simulink model "ThdRwLtStRclCmdSrvCal"  (R2024b)
settings: Solver=FixedStepDiscrete  StartTime=0.0  StopTime=10.0  FixedStep=0.01  RelTol=1e-3
undefined symbols (not defined in the file or in its folder): KeSMSwPosInvalidVal_Val, PowerMode1
settings Model: Creator=sn2xws  LastModifiedBy=sn55gm
settings SolverCC: AlgebraicLoopSolver=TrustRegion
settings DataIOCC: SaveFormat=StructureWithTime  ReturnWorkspaceOutputs=off
settings OptimizationCC: DefaultParameterBehavior=Inlined  EnhancedBackFolding=on  PassReuseOutputArgsAs=Individual arguments  ZeroExternalMemoryAtStartup=off  ZeroInternalMemoryAtStartup=off  OptimizeBlockOrder=speed  DifferentSizesBufferReuse=on  OptimizationCustomize=off  EfficientTunableParamExpr=on
settings DebuggingCC: ParameterTunabilityLossMsg=error  UnconnectedInputMsg=warning  UnconnectedOutputMsg=warning  UnconnectedLineMsg=warning  ArithmeticOperatorsInVariantConditions=warning
settings ModelReferenceCC: EnableRefExpFcnMdlSchedulingChecks=on  ModelReferenceNumInstancesAllowed=Single
settings SFSimCC: MATLABDynamicMemAlloc=off  CustomCodeUndefinedFunction=UseInterfaceOnly
settings RTWCC: Description=AUTOSAR  SystemTargetFile=autosar.tlc  GenCodeOnly=on  TemplateMakefile=ert_default_tmf  GenerateReport=on  IncludeHyperlinkInReport=on  LaunchReport=on  DataTypeReplacement=CDataTypesFixedWidth  GenerateTraceInfo=on  GenerateTraceReport=on  GenerateTraceReportSl=on  GenerateTraceReportSf=on  GenerateTraceReportEml=on  GenerateCodeMetricsReport=on  GPUComputeCapability=3.5
settings CodeAppCC: ForceParamTrailComments=on  IgnoreCustomStorageClasses=off  OperatorAnnotations=on  SimulinkDataObjDesc=on  SFDataObjDesc=on  InsertBlockDesc=on
settings STFCustomTargetCC: TargetLangStandard=C99 (ISO)  MultiwordLength=256  ParMdlRefBuildCompliant=on  CompOptLevelCompliant=on  IncludeMdlTerminateFcn=off  CombineOutputUpdateFcns=on  SuppressErrorStatus=on  ERTCustomFileBanners=on  SupportNonFinite=off  SupportComplex=off  SupportContinuousTime=off  SupportNonInlinedSFcns=off  RemoveResetFunc=on  MATLABClassNameForMDSCustomization=Simulink.SoftwareTarget.ERTCustomization  AutosarCompliant=on  UseToolchainInfoCompliant=on  LookupTableObjectStructAxisOrder=2,1,3,4,...  LUTObjectStructOrderEvenSpacing=Size,Table,Breakpoints  SystemTargetFile=autosar.tlc
settings ERTTargetCC: TargetLangStandard=C99 (ISO)  ConcurrentExecutionCompliant=off  IncludeMdlTerminateFcn=off  SuppressErrorStatus=on  SupportNonFinite=off  SupportComplex=off  ModelStepFunctionPrototypeControlCompliant=off  CPPClassGenCompliant=off  AutosarCompliant=on  LookupTableObjectStructAxisOrder=2,1,3,4,...  LUTObjectStructOrderEvenSpacing=Size,Table,Breakpoints  ERTCustomFileTemplate=example_file_process.tlc  ERTFilePackagingFormat=Compact  BooleanTrueId=TRUE  BooleanFalseId=FALSE  DynamicArrayContainerType=coder::array

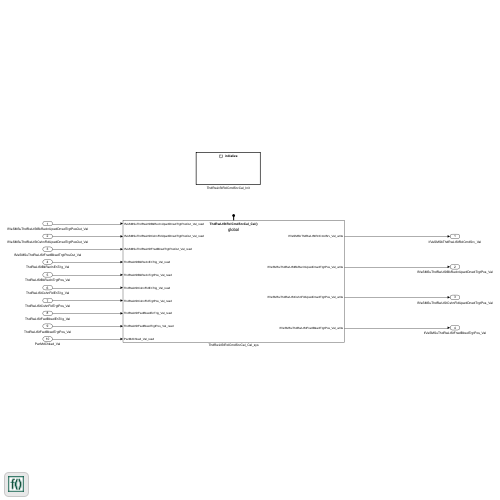
[thumbnail: Simulink's stored preview of the top-level diagram]
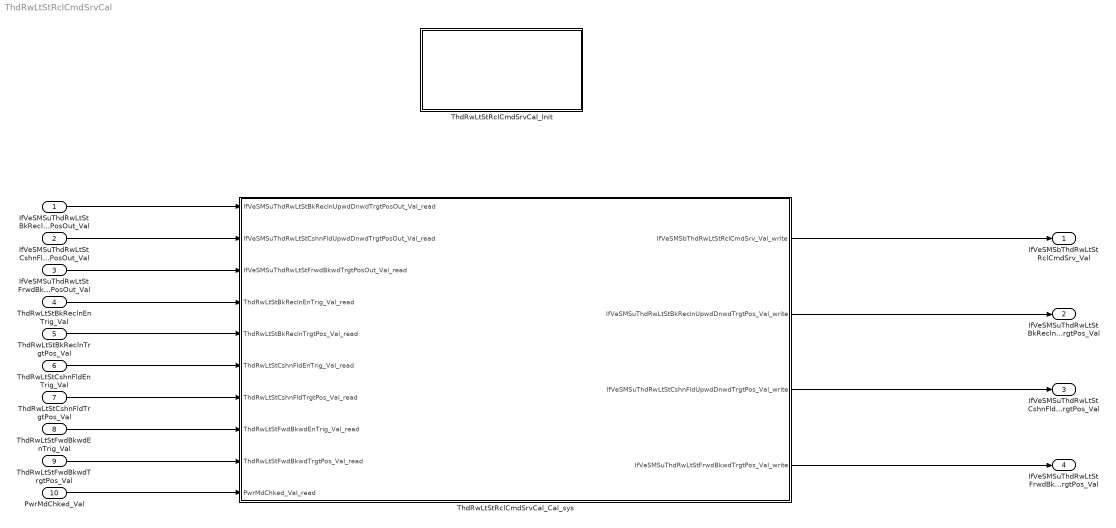
== system ThdRwLtStRclCmdSrvCal ==
  IfVeSMSuThdRwLtStBkReclnUpwdDnwdTrgtPosOut_Val : Inport  OutDataTypeStr=boolean  PortDimensions=1
  IfVeSMSuThdRwLtStCshnFldUpwdDnwdTrgtPosOut_Val : Inport  Port=2  OutDataTypeStr=boolean  PortDimensions=1
  IfVeSMSuThdRwLtStFrwdBkwdTrgtPosOut_Val : Inport  Port=3  OutDataTypeStr=boolean  PortDimensions=1
  ThdRwLtStBkReclnEnTrig_Val : Inport  Port=4  OutDataTypeStr=boolean  PortDimensions=1
  ThdRwLtStBkReclnTrgtPos_Val : Inport  Port=5  OutDataTypeStr=uint16  PortDimensions=1
  ThdRwLtStCshnFldEnTrig_Val : Inport  Port=6  OutDataTypeStr=boolean  PortDimensions=1
  ThdRwLtStCshnFldTrgtPos_Val : Inport  Port=7  OutDataTypeStr=uint16  PortDimensions=1
  ThdRwLtStFwdBkwdEnTrig_Val : Inport  Port=8  OutDataTypeStr=boolean  PortDimensions=1
  ThdRwLtStFwdBkwdTrgtPos_Val : Inport  Port=9  OutDataTypeStr=uint16  PortDimensions=1
  PwrMdChked_Val : Inport  Port=10  OutDataTypeStr=Enum: PowerMode1  PortDimensions=1
  ThdRwLtStRclCmdSrvCal_Cal_sys : Subsystem
  ThdRwLtStRclCmdSrvCal_Init : Subsystem
  IfVeSMSbThdRwLtStRclCmdSrv_Val : Outport  OutDataTypeStr=boolean  PortDimensions=1  VectorParamsAs1DForOutWhenUnconnected=off
  IfVeSMSuThdRwLtStBkReclnUpwdDnwdTrgtPos_Val : Outport  Port=2  OutDataTypeStr=uint16  PortDimensions=1  VectorParamsAs1DForOutWhenUnconnected=off
  IfVeSMSuThdRwLtStCshnFldUpwdDnwdTrgtPos_Val : Outport  Port=3  OutDataTypeStr=uint16  PortDimensions=1  VectorParamsAs1DForOutWhenUnconnected=off
  IfVeSMSuThdRwLtStFrwdBkwdTrgtPos_Val : Outport  Port=4  OutDataTypeStr=uint16  PortDimensions=1  VectorParamsAs1DForOutWhenUnconnected=off
  wires:
  IfVeSMSuThdRwLtStBkReclnUpwdDnwdTrgtPosOut_Val/1 -> ThdRwLtStRclCmdSrvCal_Cal_sys/1(IfVeSMSuThdRwLtStBkReclnUpwdDnwdTrgtPosOut_Val_read)
  IfVeSMSuThdRwLtStCshnFldUpwdDnwdTrgtPosOut_Val/1 -> ThdRwLtStRclCmdSrvCal_Cal_sys/2(IfVeSMSuThdRwLtStCshnFldUpwdDnwdTrgtPosOut_Val_read)
  IfVeSMSuThdRwLtStFrwdBkwdTrgtPosOut_Val/1 -> ThdRwLtStRclCmdSrvCal_Cal_sys/3(IfVeSMSuThdRwLtStFrwdBkwdTrgtPosOut_Val_read)
  ThdRwLtStBkReclnEnTrig_Val/1 -> ThdRwLtStRclCmdSrvCal_Cal_sys/4(ThdRwLtStBkReclnEnTrig_Val_read)
  ThdRwLtStBkReclnTrgtPos_Val/1 -> ThdRwLtStRclCmdSrvCal_Cal_sys/5(ThdRwLtStBkReclnTrgtPos_Val_read)
  ThdRwLtStCshnFldEnTrig_Val/1 -> ThdRwLtStRclCmdSrvCal_Cal_sys/6(ThdRwLtStCshnFldEnTrig_Val_read)
  ThdRwLtStCshnFldTrgtPos_Val/1 -> ThdRwLtStRclCmdSrvCal_Cal_sys/7(ThdRwLtStCshnFldTrgtPos_Val_read)
  ThdRwLtStFwdBkwdEnTrig_Val/1 -> ThdRwLtStRclCmdSrvCal_Cal_sys/8(ThdRwLtStFwdBkwdEnTrig_Val_read)
  ThdRwLtStFwdBkwdTrgtPos_Val/1 -> ThdRwLtStRclCmdSrvCal_Cal_sys/9(ThdRwLtStFwdBkwdTrgtPos_Val_read)
  ThdRwLtStRclCmdSrvCal_Cal_sys/1(IfVeSMSbThdRwLtStRclCmdSrv_Val_write) -> IfVeSMSbThdRwLtStRclCmdSrv_Val/1
  ThdRwLtStRclCmdSrvCal_Cal_sys/2(IfVeSMSuThdRwLtStBkReclnUpwdDnwdTrgtPos_Val_write) -> IfVeSMSuThdRwLtStBkReclnUpwdDnwdTrgtPos_Val/1
  ThdRwLtStRclCmdSrvCal_Cal_sys/3(IfVeSMSuThdRwLtStCshnFldUpwdDnwdTrgtPos_Val_write) -> IfVeSMSuThdRwLtStCshnFldUpwdDnwdTrgtPos_Val/1
  ThdRwLtStRclCmdSrvCal_Cal_sys/4(IfVeSMSuThdRwLtStFrwdBkwdTrgtPos_Val_write) -> IfVeSMSuThdRwLtStFrwdBkwdTrgtPos_Val/1
  PwrMdChked_Val/1 -> ThdRwLtStRclCmdSrvCal_Cal_sys/10(PwrMdChked_Val_read)

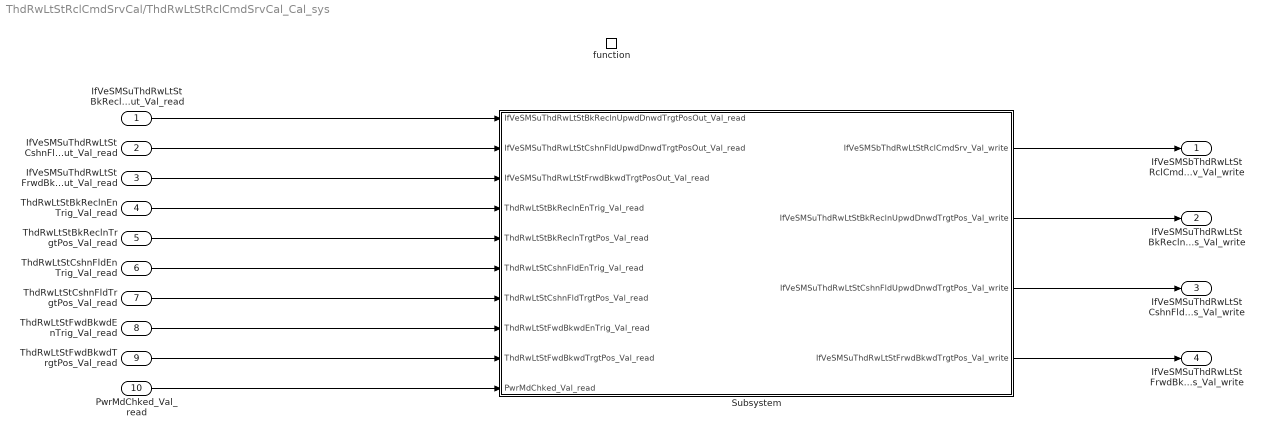
== system ThdRwLtStRclCmdSrvCal/ThdRwLtStRclCmdSrvCal_Cal_sys ==
  IfVeSMSuThdRwLtStBkReclnUpwdDnwdTrgtPosOut_Val_read : Inport
  IfVeSMSuThdRwLtStCshnFldUpwdDnwdTrgtPosOut_Val_read : Inport  Port=2
  IfVeSMSuThdRwLtStFrwdBkwdTrgtPosOut_Val_read : Inport  Port=3
  ThdRwLtStBkReclnEnTrig_Val_read : Inport  Port=4
  ThdRwLtStBkReclnTrgtPos_Val_read : Inport  Port=5
  ThdRwLtStCshnFldEnTrig_Val_read : Inport  Port=6
  ThdRwLtStCshnFldTrgtPos_Val_read : Inport  Port=7
  ThdRwLtStFwdBkwdEnTrig_Val_read : Inport  Port=8
  ThdRwLtStFwdBkwdTrgtPos_Val_read : Inport  Port=9
  PwrMdChked_Val_read : Inport  Port=10
  function : TriggerPort  TriggerType=function-call  IsSimulinkFunction=on  FunctionName=ThdRwLtStRclCmdSrvCal_Cal  VariantControl=(inherit)
  Subsystem : Subsystem
  IfVeSMSbThdRwLtStRclCmdSrv_Val_write : Outport  VectorParamsAs1DForOutWhenUnconnected=off
      settings: EnsureOutportIsVirtual=on
  IfVeSMSuThdRwLtStBkReclnUpwdDnwdTrgtPos_Val_write : Outport  Port=2  VectorParamsAs1DForOutWhenUnconnected=off
      settings: EnsureOutportIsVirtual=on
  IfVeSMSuThdRwLtStCshnFldUpwdDnwdTrgtPos_Val_write : Outport  Port=3  VectorParamsAs1DForOutWhenUnconnected=off
      settings: EnsureOutportIsVirtual=on
  IfVeSMSuThdRwLtStFrwdBkwdTrgtPos_Val_write : Outport  Port=4  VectorParamsAs1DForOutWhenUnconnected=off
      settings: EnsureOutportIsVirtual=on
  wires:
  Subsystem/1(IfVeSMSbThdRwLtStRclCmdSrv_Val_write) -> IfVeSMSbThdRwLtStRclCmdSrv_Val_write/1
  Subsystem/4(IfVeSMSuThdRwLtStFrwdBkwdTrgtPos_Val_write) -> IfVeSMSuThdRwLtStFrwdBkwdTrgtPos_Val_write/1
  Subsystem/3(IfVeSMSuThdRwLtStCshnFldUpwdDnwdTrgtPos_Val_write) -> IfVeSMSuThdRwLtStCshnFldUpwdDnwdTrgtPos_Val_write/1
  Subsystem/2(IfVeSMSuThdRwLtStBkReclnUpwdDnwdTrgtPos_Val_write) -> IfVeSMSuThdRwLtStBkReclnUpwdDnwdTrgtPos_Val_write/1
  IfVeSMSuThdRwLtStBkReclnUpwdDnwdTrgtPosOut_Val_read/1 -> Subsystem/1(IfVeSMSuThdRwLtStBkReclnUpwdDnwdTrgtPosOut_Val_read)
  IfVeSMSuThdRwLtStCshnFldUpwdDnwdTrgtPosOut_Val_read/1 -> Subsystem/2(IfVeSMSuThdRwLtStCshnFldUpwdDnwdTrgtPosOut_Val_read)
  IfVeSMSuThdRwLtStFrwdBkwdTrgtPosOut_Val_read/1 -> Subsystem/3(IfVeSMSuThdRwLtStFrwdBkwdTrgtPosOut_Val_read)
  ThdRwLtStBkReclnEnTrig_Val_read/1 -> Subsystem/4(ThdRwLtStBkReclnEnTrig_Val_read)
  ThdRwLtStBkReclnTrgtPos_Val_read/1 -> Subsystem/5(ThdRwLtStBkReclnTrgtPos_Val_read)
  ThdRwLtStCshnFldEnTrig_Val_read/1 -> Subsystem/6(ThdRwLtStCshnFldEnTrig_Val_read)
  ThdRwLtStCshnFldTrgtPos_Val_read/1 -> Subsystem/7(ThdRwLtStCshnFldTrgtPos_Val_read)
  ThdRwLtStFwdBkwdEnTrig_Val_read/1 -> Subsystem/8(ThdRwLtStFwdBkwdEnTrig_Val_read)
  ThdRwLtStFwdBkwdTrgtPos_Val_read/1 -> Subsystem/9(ThdRwLtStFwdBkwdTrgtPos_Val_read)
  PwrMdChked_Val_read/1 -> Subsystem/10(PwrMdChked_Val_read)

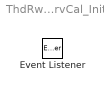
== system ThdRwLtStRclCmdSrvCal/ThdRwLtStRclCmdSrvCal_Init ==
  Event Listener : EventListener  EventName=reset

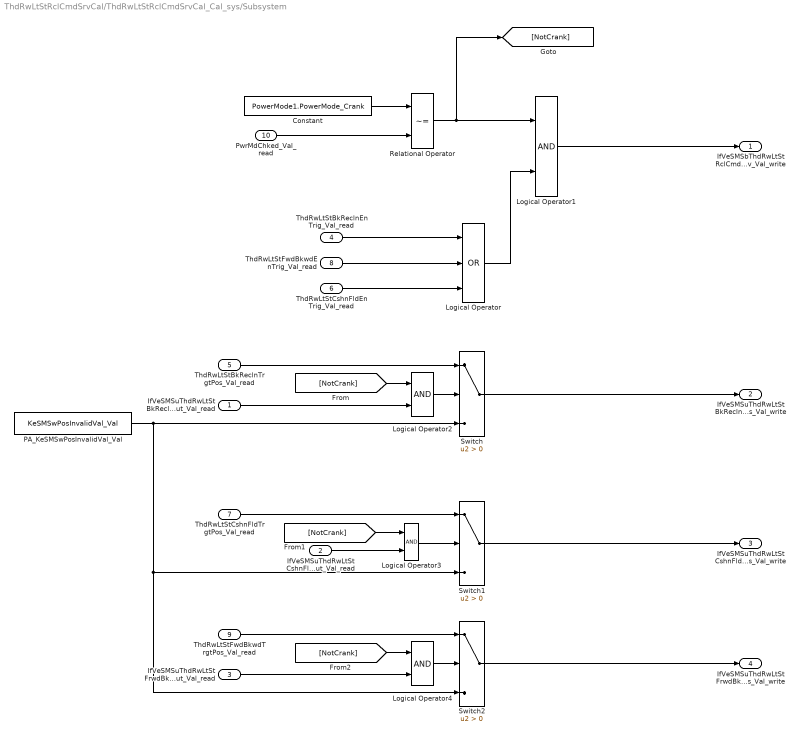
== system ThdRwLtStRclCmdSrvCal/ThdRwLtStRclCmdSrvCal_Cal_sys/Subsystem ==
  IfVeSMSuThdRwLtStBkReclnUpwdDnwdTrgtPosOut_Val_read : Inport
  IfVeSMSuThdRwLtStCshnFldUpwdDnwdTrgtPosOut_Val_read : Inport  Port=2
  IfVeSMSuThdRwLtStFrwdBkwdTrgtPosOut_Val_read : Inport  Port=3
  ThdRwLtStBkReclnEnTrig_Val_read : Inport  Port=4
  ThdRwLtStBkReclnTrgtPos_Val_read : Inport  Port=5
  ThdRwLtStCshnFldEnTrig_Val_read : Inport  Port=6
  ThdRwLtStCshnFldTrgtPos_Val_read : Inport  Port=7
  ThdRwLtStFwdBkwdEnTrig_Val_read : Inport  Port=8
  ThdRwLtStFwdBkwdTrgtPos_Val_read : Inport  Port=9
  PwrMdChked_Val_read : Inport  Port=10
  Constant : Constant  Value=PowerMode1.PowerMode_Crank  OutDataTypeStr=Enum: PowerMode1
  Logical Operator : Logic  Operator=OR  Inputs=3  AllPortsSameDT=off  OutDataTypeStr=boolean
  Logical Operator{1..4} (4 alike) : Logic  AllPortsSameDT=off  OutDataTypeStr=boolean
  PA_KeSMSwPosInvalidVal_Val : Constant  Value=KeSMSwPosInvalidVal_Val
  Relational Operator : RelationalOperator  Operator=~=  OutDataTypeStr=boolean  RndMeth=Simplest  InputSameDT=off
  Switch : Switch  Criteria=u2 > Threshold  SaturateOnIntegerOverflow=off  InputSameDT=off
  Switch1 : Switch  Criteria=u2 > Threshold  SaturateOnIntegerOverflow=off  InputSameDT=off
  Switch2 : Switch  Criteria=u2 > Threshold  SaturateOnIntegerOverflow=off  InputSameDT=off
  IfVeSMSbThdRwLtStRclCmdSrv_Val_write : Outport  VectorParamsAs1DForOutWhenUnconnected=off
      settings: EnsureOutportIsVirtual=on
  IfVeSMSuThdRwLtStBkReclnUpwdDnwdTrgtPos_Val_write : Outport  Port=2  VectorParamsAs1DForOutWhenUnconnected=off
      settings: EnsureOutportIsVirtual=on
  IfVeSMSuThdRwLtStCshnFldUpwdDnwdTrgtPos_Val_write : Outport  Port=3  VectorParamsAs1DForOutWhenUnconnected=off
      settings: EnsureOutportIsVirtual=on
  IfVeSMSuThdRwLtStFrwdBkwdTrgtPos_Val_write : Outport  Port=4  VectorParamsAs1DForOutWhenUnconnected=off
      settings: EnsureOutportIsVirtual=on
  wires:
  ThdRwLtStBkReclnEnTrig_Val_read/1 -> Logical Operator/1
  ThdRwLtStFwdBkwdTrgtPos_Val_read/1 -> Switch2/1
  PA_KeSMSwPosInvalidVal_Val/1 -> Switch2/3, Switch1/3, Switch/3
  ThdRwLtStCshnFldTrgtPos_Val_read/1 -> Switch1/1
  Switch/1 -> IfVeSMSuThdRwLtStBkReclnUpwdDnwdTrgtPos_Val_write/1
  ThdRwLtStCshnFldEnTrig_Val_read/1 -> Logical Operator/3
  ThdRwLtStFwdBkwdEnTrig_Val_read/1 -> Logical Operator/2
  Switch1/1 -> IfVeSMSuThdRwLtStCshnFldUpwdDnwdTrgtPos_Val_write/1
  Switch2/1 -> IfVeSMSuThdRwLtStFrwdBkwdTrgtPos_Val_write/1
  ThdRwLtStBkReclnTrgtPos_Val_read/1 -> Switch/1
  Relational Operator/1 -> [NotCrank], Logical Operator1/1
  Constant/1 -> Relational Operator/1
  PwrMdChked_Val_read/1 -> Relational Operator/2
  Logical Operator/1 -> Logical Operator1/2
  Logical Operator1/1 -> IfVeSMSbThdRwLtStRclCmdSrv_Val_write/1
  Logical Operator2/1 -> Switch/2
  IfVeSMSuThdRwLtStBkReclnUpwdDnwdTrgtPosOut_Val_read/1 -> Logical Operator2/2
  [NotCrank] -> Logical Operator2/1
  Logical Operator4/1 -> Switch2/2
  IfVeSMSuThdRwLtStFrwdBkwdTrgtPosOut_Val_read/1 -> Logical Operator4/2
  [NotCrank] -> Logical Operator4/1
  [NotCrank] -> Logical Operator3/1
  IfVeSMSuThdRwLtStCshnFldUpwdDnwdTrgtPosOut_Val_read/1 -> Logical Operator3/2
  Logical Operator3/1 -> Switch1/2
